simulink model "equations_dyn_snchrone_triphase"  (R2018b)
settings: Solver=VariableStepAuto  StartTime=0.0  StopTime=100  RelTol=1e-3
values from neighbouring files (symbols this model uses):
  alpha = 1    [Poteau_main.m]
  ca = 0.18    [Poteau_main.m]
  g = 9.81    [Poteau_main.m]
  Lambdam = 0.0744    [Poteau_main.m]
  Ls = 0.0021    [Poteau_main.m]
  M = 92    [Poteau_main.m]
  Np = 52    [Poteau_main.m]
  Rs = 0.124    [Poteau_main.m]
  Rw = 0.33    [Poteau_main.m]
  s = tan(inc)    [Poteau_main.m]
libraries: simulink x2
settings Model: Creator=poteaum  LastModifiedBy=poteaum

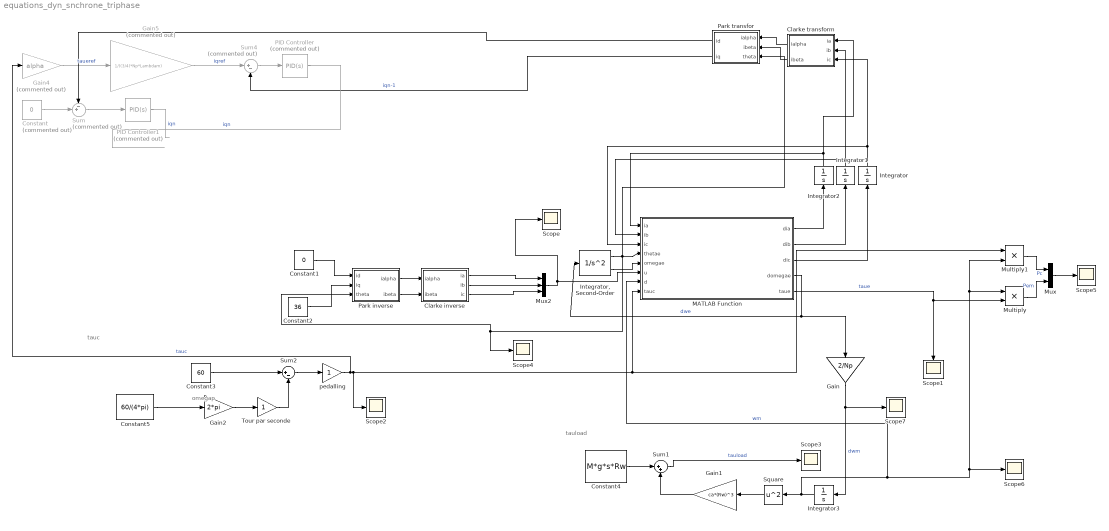
== system equations_dyn_snchrone_triphase ==
  note: omegap
  note: tauc
  note: tauload
  Clarke inverse : MATLAB Function  TreatAsAtomicUnit=on
  "Clarke transform " : MATLAB Function  TreatAsAtomicUnit=on
  Constant : Constant  Commented=on  Value=0
  Constant1 : Constant  Value=0
  Constant2 : Constant  Value=36
  Constant3 : Constant  Value=60
  Constant4 : Constant  Value=M*g*s*Rw
  Constant5 : Constant  Value=60/(4*pi)
  Gain : Gain  Gain=2/Np
  Gain1 : Gain  Gain=ca*(Rw)^3
  Gain2 : Gain  Gain=2*pi
  Gain4 : Gain  Commented=on  Gain=alpha
  Gain5 : Gain  Commented=on  Gain=1/((3/4)*Np*Lambdam)
  Integrator{,1..3} (4 alike) : Integrator
  "Integrator, Second-Order" : SecondOrderIntegrator
  MATLAB Function : MATLAB Function  TreatAsAtomicUnit=on
  Multiply : Product
  Multiply1 : Product
  Mux : Mux  Inputs=2
  Mux2 : Mux  Inputs=3
  PID Controller : simulink/Continuous/PID Controller  Commented=on  Controller=PID  Form=Parallel  TimeDomain=Continuous-time  SampleTime=-1  IntegratorMethod=Forward Euler  FilterMethod=Forward Euler  ControllerParametersSource=internal  P=2*Rs-Rs  I=Rs^2/Ls  D=1.6  UseFilter=on  N=100  TunerSelectOption=Transfer Function Based (PID Tuner App)  InitialConditionSource=internal  InitialConditionForIntegrator=0  InitialConditionForFilter=0  DifferentiatorICPrevScaledInput=0  ExternalReset=none  TrackingMode=off  Kt=1  LimitOutput=off  UpperSaturationLimit=inf  LowerSaturationLimit=-inf  LinearizeAsGain=on  AntiWindupMode=none  Kb=1  POutMin=[]  POutMax=[]  IOutMin=[]  IOutMax=[]  DOutMin=[]  DOutMax=[]  NOutMin=[]  NOutMax=[]  SumOutMin=[]  SumOutMax=[]  SaturationOutMin=[]  SaturationOutMax=[]  PParamMin=[]  PParamMax=[]  IParamMin=[]  IParamMax=[]  DParamMin=[]  DParamMax=[]  NParamMin=[]  NParamMax=[]  KbParamMin=[]  KbParamMax=[]  KtParamMin=[]  KtParamMax=[]  KbOutMin=[]  KbOutMax=[]  KtOutMin=[]  KtOutMax=[]  IntegratorOutMin=[]  IntegratorOutMax=[]  FilterOutMin=[]  FilterOutMax=[]  SumI1OutMin=[]  SumI1OutMax=[]  SumI2OutMin=[]  SumI2OutMax=[]  SumI3OutMin=[]  SumI3OutMax=[]  SumI4OutMin=[]  SumI4OutMax=[]  SumDOutMin=[]  SumDOutMax=[]  DifferentiatorOutMin=[]  DifferentiatorOutMax=[]  FilterDiffOutCoefMin=[]  FilterDiffOutCoefMax=[]  ReciprocalOutMin=[]  ReciprocalOutMax=[]  SumDenOutMin=[]  SumDenOutMax=[]  SumNumOutMin=[]  SumNumOutMax=[]  DivideOutMin=[]  DivideOutMax=[]  IntegratorContinuousStateAttributes=''  IntegratorStateMustResolveToSignalObject=off  IntegratorRTWStateStorageClass=Auto  FilterContinuousStateAttributes=''  FilterStateMustResolveToSignalObject=off  FilterRTWStateStorageClass=Auto  ParallelPVariant=InternalParameters  IdealPVariant=Disabled  IVariant=InternalParameters  DVariant=InternalParameters  IntegratorVariant=Continuous  SatVariant=Disabled  AWVariant=Passthrough  PCopyVariant=Disabled  TRVariant=Disabled  FdbkBlocksVariant=Forward  IdealPFdbkVariant=Disabled  SatFdbkVariant=Disabled  DerivativeFilterVariant=ContFilter  NVariant=InternalParameters  NCopyVariant=Disabled  FilterICVariant=InternalICsFilter  IntegratorICVariant=InternalICs  ExternalResetVariant=Disabled  TRSumVariant=Passthrough  SumFdbkVariant=Disabled  SumVariant=Sum_PID
  PID Controller1 : simulink/Continuous/PID Controller  Commented=on  Controller=PID  Form=Parallel  TimeDomain=Continuous-time  SampleTime=-1  IntegratorMethod=Forward Euler  FilterMethod=Forward Euler  ControllerParametersSource=internal  P=2*Rs-Rs  I=Rs^2/Ls  D=1.6  UseFilter=on  N=100  TunerSelectOption=Transfer Function Based (PID Tuner App)  InitialConditionSource=internal  InitialConditionForIntegrator=0  InitialConditionForFilter=0  DifferentiatorICPrevScaledInput=0  ExternalReset=none  TrackingMode=off  Kt=1  LimitOutput=off  UpperSaturationLimit=inf  LowerSaturationLimit=-inf  LinearizeAsGain=on  AntiWindupMode=none  Kb=1  POutMin=[]  POutMax=[]  IOutMin=[]  IOutMax=[]  DOutMin=[]  DOutMax=[]  NOutMin=[]  NOutMax=[]  SumOutMin=[]  SumOutMax=[]  SaturationOutMin=[]  SaturationOutMax=[]  PParamMin=[]  PParamMax=[]  IParamMin=[]  IParamMax=[]  DParamMin=[]  DParamMax=[]  NParamMin=[]  NParamMax=[]  KbParamMin=[]  KbParamMax=[]  KtParamMin=[]  KtParamMax=[]  KbOutMin=[]  KbOutMax=[]  KtOutMin=[]  KtOutMax=[]  IntegratorOutMin=[]  IntegratorOutMax=[]  FilterOutMin=[]  FilterOutMax=[]  SumI1OutMin=[]  SumI1OutMax=[]  SumI2OutMin=[]  SumI2OutMax=[]  SumI3OutMin=[]  SumI3OutMax=[]  SumI4OutMin=[]  SumI4OutMax=[]  SumDOutMin=[]  SumDOutMax=[]  DifferentiatorOutMin=[]  DifferentiatorOutMax=[]  FilterDiffOutCoefMin=[]  FilterDiffOutCoefMax=[]  ReciprocalOutMin=[]  ReciprocalOutMax=[]  SumDenOutMin=[]  SumDenOutMax=[]  SumNumOutMin=[]  SumNumOutMax=[]  DivideOutMin=[]  DivideOutMax=[]  IntegratorContinuousStateAttributes=''  IntegratorStateMustResolveToSignalObject=off  IntegratorRTWStateStorageClass=Auto  FilterContinuousStateAttributes=''  FilterStateMustResolveToSignalObject=off  FilterRTWStateStorageClass=Auto  ParallelPVariant=InternalParameters  IdealPVariant=Disabled  IVariant=InternalParameters  DVariant=InternalParameters  IntegratorVariant=Continuous  SatVariant=Disabled  AWVariant=Passthrough  PCopyVariant=Disabled  TRVariant=Disabled  FdbkBlocksVariant=Forward  IdealPFdbkVariant=Disabled  SatFdbkVariant=Disabled  DerivativeFilterVariant=ContFilter  NVariant=InternalParameters  NCopyVariant=Disabled  FilterICVariant=InternalICsFilter  IntegratorICVariant=InternalICs  ExternalResetVariant=Disabled  TRSumVariant=Passthrough  SumFdbkVariant=Disabled  SumVariant=Sum_PID
  "Park inverse " : MATLAB Function  TreatAsAtomicUnit=on
  "Park transfor " : MATLAB Function  TreatAsAtomicUnit=on
  Scope{,1..7} (8 alike) : Scope
  Square : Math  Operator=square  OutputSignalType=real  SaturateOnIntegerOverflow=on
  Sum : Sum  Commented=on  Inputs=-+|
  Sum1 : Sum  Inputs=|++
  Sum2 : Sum  Inputs=|+-
  Sum4 : Sum  Commented=on  Inputs=|+-
  Tour par seconde : Gain
  "pedalling " : Gain
  wires:
  MATLAB Function/1(dia) -> Integrator2/1
  MATLAB Function/2(dib) -> Integrator1/1
  MATLAB Function/3(dic) -> Integrator/1
  "Integrator, Second-Order"/1 -> Scope4/1, "Park inverse "/3(theta), "Park transfor "/3(theta), MATLAB Function/4(thetae)
  "Integrator, Second-Order"/2 -> MATLAB Function/5(omegae)
  Clarke inverse/3(ic) -> Mux2/3
  Mux2/1 -> Scope/1, MATLAB Function/6(u)
  Clarke inverse/1(ia) -> Mux2/1
  Clarke inverse/2(ib) -> Mux2/2
  "Park inverse "/2(ibeta) -> Clarke inverse/2(ibeta)
  "Park inverse "/1(ialpha) -> Clarke inverse/1(ialpha)
  Constant3/1 -> Sum2/1
  Sum2/1 -> "pedalling "/1
  Tour par seconde/1 -> Sum2/2
  Constant4/1 -> Sum1/1
  Integrator3/1 -> MATLAB Function/7(d), Scope6/1, Multiply1/2, Multiply/1, Square/1  "wm"
  Gain1/1 -> Sum1/2
  Square/1 -> Gain1/1
  MATLAB Function/4(domegae) -> Gain/1, "Integrator, Second-Order"/1  "dwe"
  Constant5/1 -> Gain2/1
  Gain2/1 -> Tour par seconde/1
  Gain/1 -> Scope7/1, Integrator3/1  "dwm"
  MATLAB Function/5(taue) -> Scope1/1, Multiply/2  "taue"
  "pedalling "/1 -> Multiply1/1, MATLAB Function/8(tauc), Scope2/1, Gain4/1  "tauc"
  Sum1/1 -> Scope3/1  "tauload"
  "Clarke transform "/1(ialpha) -> "Park transfor "/1(ialpha)
  "Clarke transform "/2(ibeta) -> "Park transfor "/2(ibeta)
  Integrator2/1 -> MATLAB Function/1(ia), "Clarke transform "/1(ia)
  Integrator1/1 -> "Clarke transform "/2(ib), MATLAB Function/2(ib)
  Integrator/1 -> MATLAB Function/3(ic), "Clarke transform "/3(ic)
  Gain4/1 -> Gain5/1  "taueref"
  Sum4/1 -> PID Controller/1
  Gain5/1 -> Sum4/1  "iqref"
  "Park transfor "/2(iq) -> Sum4/2  "iqn-1"
  PID Controller/1 -> ?  "iqn"
  Constant/1 -> Sum/2
  "Park transfor "/1(id) -> Sum/1
  Sum/1 -> PID Controller1/1
  Multiply1/1 -> Mux/1  "Pc"
  Multiply/1 -> Mux/2  "Pem"
  Mux/1 -> Scope5/1
  PID Controller1/1 -> ?  "iqn"
  Constant2/1 -> "Park inverse "/2(iq)
  Constant1/1 -> "Park inverse "/1(id)

== matlab function equations_dyn_snchrone_triphase/Clarke inverse ==
  data: ialpha input; ia output; ibeta input; ib output; ic output
function [ia,ib,ic]= fcn(ialpha,ibeta)
I = [ialpha; ibeta; 0];
M_C=[1 0 0;1/sqrt(3) 2/sqrt(3) 0; 1 1 1];
solu=inv(M_C)*I;
ia = solu(1);
ib=solu(2);
ic= solu(3);
end

== matlab function equations_dyn_snchrone_triphase/MATLAB Function ==
  data: ia input size=1; ib input size=1; ic input size=1; thetae input size=1; omegae input size=1; u input size=3; dia output size=1; d input size=1; dib output size=1; dic output size=1; domegae output size=1; tauc input size=1; taue output
function [dia, dib, dic, domegae, taue] = DynamiqueSynchroneTriphase(ia,ib, ic, thetae, omegae, u, d, tauc)
Rs=0.124;   %R STATOR
Ls=0.0021;   %L Stator
Lambdam=0.0744; %Flux magnétique
Np=52;  %Nb poles
Jm=0.0028;  %Moment d'inertie moteur
M=92;   %Masse totale
Rw=0.33;
Jt=M*Rw*Rw;


va = u(1); vb = u(2); vc = u(3);
dia = va/Ls - (Rs/Ls) * ia + (Lambdam/Ls) * omegae*sin(thetae);
dib = vb/Ls - (Rs/Ls) * ib + (Lambdam/Ls) * omegae*sin(thetae-(2*pi/3));
dic = vc/Ls - (Rs/Ls) * ic + (Lambdam/Ls) * omegae*sin(thetae+(2*pi/3));
taue = (Np / 2) * (ia * Lambdam * (-sin(thetae)) + ib * Lambdam * (-sin(thetae-(2*pi/3))) + ic * Lambdam * (-sin(thetae+(2*pi/3))));
domegae = (Np/(Jt * 2)) * (taue - d + tauc);

== matlab function equations_dyn_snchrone_triphase/Clarke transform  ==
  data: ia input; ialpha output; ib input; ic input; ibeta output
function [ialpha,ibeta]= fcn(ia,ib,ic)
I =[ ia;ib;ic];
M_C=[1 0 0;1/sqrt(3) 2/sqrt(3) 0; 1 1 1];
solu=(M_C)*I;
ialpha= solu(1);
ibeta=solu(2);
end

== matlab function equations_dyn_snchrone_triphase/Park inverse  ==
  data: id input; ialpha output; iq input; ibeta output; theta input
function [ialpha,ibeta]= fcn(id,iq,theta)
I=[id; iq]
M_P=[cos(theta) sin(theta); -sin(theta) cos(theta)];
solu=inv(M_P)*I;
ialpha = solu(1);
ibeta=solu(2);
end

== matlab function equations_dyn_snchrone_triphase/Park transfor  ==
  data: ialpha input; id output; ibeta input; iq output; theta input
function [id,iq]= fcn(ialpha,ibeta,theta)

I=[ialpha;ibeta];
M_P=[cos(theta) sin(theta); -sin(theta) cos(theta)];
solu=M_P*I;
id=solu(1);
iq=solu(2);

end
